simulink model "dynamiczny_ciagly_for_print"  (R2020a)
settings: Solver=VariableStepAuto  StartTime=0.0  StopTime=10.0  RelTol=1e-3
values from neighbouring files (symbols this model uses):
  a1 = 0.56    [init_values.m]
  a2 = -0.8    [init_values.m]
  a3 = -0.25    [init_values.m]
  a4 = 0.2    [init_values.m]
  K = 4    [init_values.m]
  T1 = 4    [init_values.m]
  T2 = 10    [init_values.m]
settings Model: Creator=jakub  LastModifiedBy=jakub

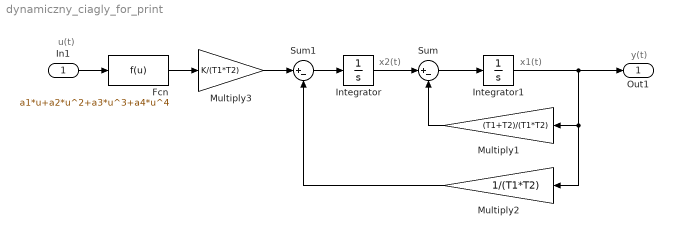
== system dynamiczny_ciagly_for_print ==
  note: u(t)
  note: y(t)
  note: x1(t)
  note: x2(t)
  In1 : Inport
  Fcn : Fcn  Expr=a1*u+a2*u^2+a3*u^3+a4*u^4
  Integrator : Integrator  ZeroCross=off
  Integrator1 : Integrator  ZeroCross=off
  Multiply1 : Gain  Gain=(T1+T2)/(T1*T2)
  Multiply2 : Gain  Gain=1/(T1*T2)
  Multiply3 : Gain  Gain=K/(T1*T2)
  Sum : Sum  Inputs=|+-
  Sum1 : Sum  Inputs=|+-
  Out1 : Outport
  wires:
  Integrator1/1 -> Multiply2/1, Multiply1/1, Out1/1
  Multiply1/1 -> Sum/2
  Integrator/1 -> Sum/1
  Sum/1 -> Integrator1/1
  Multiply2/1 -> Sum1/2
  Sum1/1 -> Integrator/1
  Multiply3/1 -> Sum1/1
  In1/1 -> Fcn/1
  Fcn/1 -> Multiply3/1
